simulink model "Ex2s"  (R2025a)
settings: Solver=VariableStepAuto  StartTime=0.0  StopTime=10.0  RelTol=1e-3
undefined symbols (not defined in the file): DiscIntNeverNeededParam

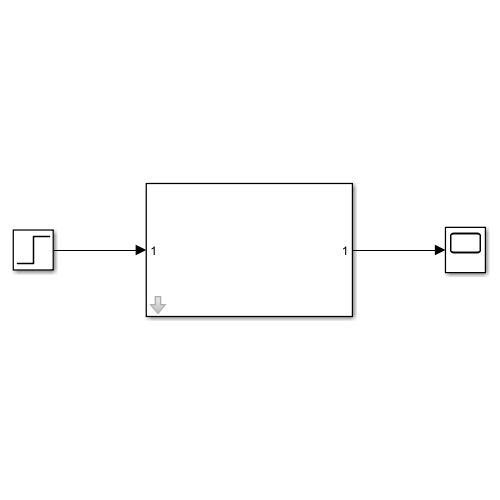
[thumbnail: Simulink's stored preview of the top-level diagram]
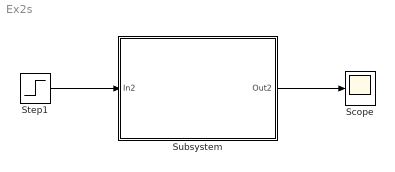
== system Ex2s ==
  Scope : Scope
      settings: ActiveDisplayYMinimum=-0.12628038359091592  ActiveDisplayYMaximum=1.1365234523182435
  Step1 : Step  SampleTime=0
  Subsystem : Subsystem  mask{SampleTime=0.1}
      mask prompts: SampleTime "Sample Time"
  wires:
  Subsystem/1(Out2) -> Scope/1
  Step1/1 -> Subsystem/1(In2)

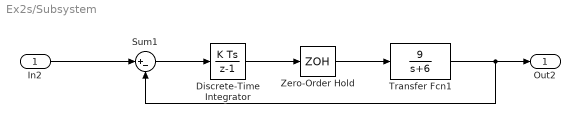
== system Ex2s/Subsystem ==
  In2 : Inport
  Discrete-Time Integrator : DiscreteIntegrator  SampleTime=-1  ICPrevOutput=DiscIntNeverNeededParam  ICPrevScaledInput=DiscIntNeverNeededParam
  Sum1 : Sum  Inputs=|+-  SampleTime=SampleTime
  Transfer Fcn1 : TransferFcn  Numerator=[9]  Denominator=[1 6]
  Zero-Order Hold : ZeroOrderHold  SampleTime=-1
  Out2 : Outport
  wires:
  Zero-Order Hold/1 -> Transfer Fcn1/1
  Transfer Fcn1/1 -> Out2/1, Sum1/2
  Discrete-Time Integrator/1 -> Zero-Order Hold/1
  Sum1/1 -> Discrete-Time Integrator/1
  In2/1 -> Sum1/1
